simulink model "threephaseunipolar"  (Simulink 8.3)
settings: Solver=ode45  StartTime=0.0  StopTime=0.5  RelTol=1e-3
libraries: powerlib x13, simulink x3
settings Model: Creator=Singhal  LastModifiedBy=Singhal
settings OptimizationCC: ExpressionDepthLimit=2147483647
settings DebuggingCC: FcnCallInpInsideContextMsg=UseLocalSettings

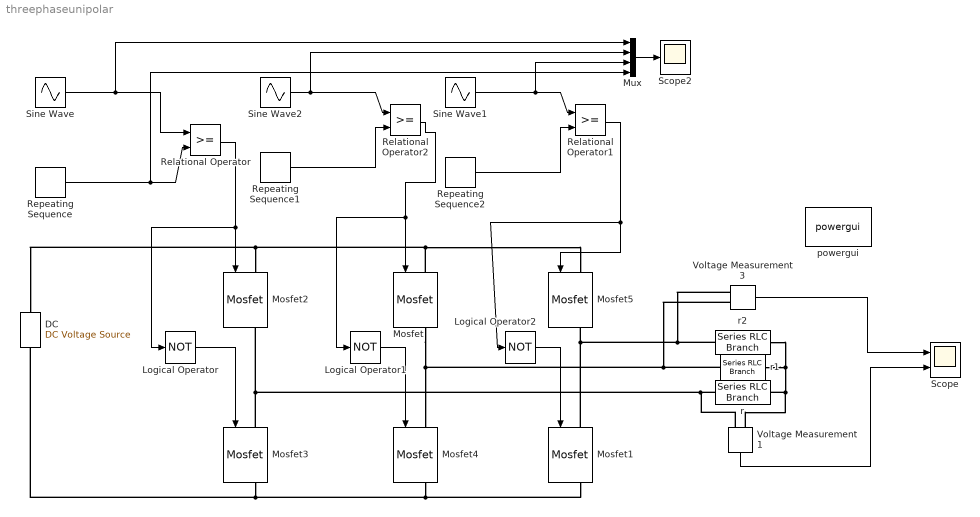
== system threephaseunipolar ==
  DC : powerlib/Electrical Sources/DC Voltage Source  Amplitude=100  Measurements=None
  Logical Operator : Logic  Operator=NOT  AllPortsSameDT=off  OutDataTypeStr=boolean
  Logical Operator1 : Logic  Operator=NOT  AllPortsSameDT=off  OutDataTypeStr=boolean
  Logical Operator2 : Logic  Operator=NOT  AllPortsSameDT=off  OutDataTypeStr=boolean
  Mosfet{,1..5} (6 alike) : powerlib/Power Electronics/Mosfet  Ron=0.1  Lon=0  Rd=0.01  Vfd=0  IC=0  Rs=1e5  Cs=inf  Measurements=on
  Mux : Mux
  Relational Operator : RelationalOperator  OutDataTypeStr=boolean
  Relational Operator1 : RelationalOperator  OutDataTypeStr=boolean
  Relational Operator2 : RelationalOperator  OutDataTypeStr=boolean
  Repeating Sequence : simulink/Sources/Repeating Sequence  rep_seq_t=[0 0.005/20 0.01/20 0.015/20 0.02/20]  rep_seq_y=[0 1 0 -1 0]
  Repeating Sequence1 : simulink/Sources/Repeating Sequence  rep_seq_t=[0 0.005/20 0.01/20 0.015/20 0.02/20]  rep_seq_y=[0 1 0 -1 0]
  Repeating Sequence2 : simulink/Sources/Repeating Sequence  rep_seq_t=[0 0.005/20 0.01/20 0.015/20 0.02/20]  rep_seq_y=[0 1 0 -1 0]
  Scope : Scope  NumInputPorts=2
      settings: YMin=-100~-5  YMax=100~5
  Scope2 : Scope
      settings: YMin=-100  YMax=100  SaveName=ScopeData2
  Sine Wave : Sin  Frequency=50*2*3.14  SampleTime=0
  Sine Wave1 : Sin  Frequency=50*2*3.14  Phase=-3.14*(4/3)  SampleTime=0
  Sine Wave2 : Sin  Frequency=50*2*3.14  Phase=-3.14*(2/3)  SampleTime=0
  Voltage Measurement1 : powerlib/Measurements/Voltage Measurement  PhasorSimulation=off  OutputType=Complex  PSBequivalent=0
  Voltage Measurement3 : powerlib/Measurements/Voltage Measurement  PhasorSimulation=off  OutputType=Complex  PSBequivalent=0
  powergui : powerlib/powergui  Priority=1  SimulationMode=Discrete  SolverType=Tustin  SampleTime=50e-6  frequency=60  SPID=off  DisableSnubberDevices=off  DisableRonSwitches=off  DisableVfSwitches=off  SwTol=0  Interpol=off  DisplayEquations=off  Ts=0  methode=off  frequencyindice=0  Pbase=100e6  ErrMax=1e-4  Iterations=50  UnitsV=kV  UnitsW=MW  FunctionMessages=off  echomessages=off  HookPort=off  EnableUseOfTLC=off  x0status=blocks  RestoreLinks=warning  ResistiveCurrentMeasurement=off  Frange=[0:2:500]  Ylog=off  Xlog=on  ShowGrid=off  save=off  variable=ZData  structure=ScopeData  ZoomFFT=on  StartTime=0.0  cycles=1  DisplayStyle=2  fundamental=50  FreqAxis=off  MaxFrequency=1000  frequencyindicesteady=1  RmsSteady=1  display=off
  r : powerlib/Elements/Series RLC Branch  LConnTagsString=__new0  RConnTagsString=__new0  BranchType=R  Resistance=1  Inductance=1e-3  SetiL0=off  InitialCurrent=0  Capacitance=1e-6  Setx0=off  InitialVoltage=0  Measurements=None
  r1 : powerlib/Elements/Series RLC Branch  LConnTagsString=__new0  RConnTagsString=__new0  BranchType=R  Resistance=1  Inductance=1e-3  SetiL0=off  InitialCurrent=0  Capacitance=1e-6  Setx0=off  InitialVoltage=0  Measurements=None
  r2 : powerlib/Elements/Series RLC Branch  LConnTagsString=__new0  RConnTagsString=__new0  BranchType=R  Resistance=1  Inductance=1e-3  SetiL0=off  InitialCurrent=0  Capacitance=1e-6  Setx0=off  InitialVoltage=0  Measurements=None
  wires:
  Sine Wave/1 -> Relational Operator/1, Mux/1
  Repeating Sequence/1 -> Relational Operator/2, Mux/4
  Logical Operator/1 -> Mosfet3/1
  Repeating Sequence2/1 -> Relational Operator1/2
  Sine Wave1/1 -> Relational Operator1/1, Mux/3
  Logical Operator1/1 -> Mosfet4/1
  Logical Operator2/1 -> Mosfet1/1
  Repeating Sequence1/1 -> Relational Operator2/2
  Sine Wave2/1 -> Relational Operator2/1, Mux/2
  Relational Operator1/1 -> Mosfet5/1, Logical Operator2/1
  Relational Operator2/1 -> Mosfet/1, Logical Operator1/1
  Relational Operator/1 -> Mosfet2/1, Logical Operator/1
  Mux/1 -> Scope2/1
  Voltage Measurement1/1 -> Scope/2
  Voltage Measurement3/1 -> Scope/1
  connections:
  Mosfet/LConn1 -- DC/RConn1 -- Mosfet2/LConn1 -- Mosfet5/LConn1
  Mosfet4/RConn1 -- DC/LConn1 -- Mosfet3/RConn1 -- Mosfet1/RConn1
  Mosfet1/LConn1 -- Voltage Measurement3/LConn1 -- r2/LConn1 -- Mosfet5/RConn1
  Mosfet/RConn1 -- r1/RConn1 -- Voltage Measurement3/LConn2 -- Mosfet4/LConn1
  Mosfet3/LConn1 -- Voltage Measurement1/LConn1 -- r/LConn1 -- Mosfet2/RConn1
  r2/RConn1 -- r1/LConn1 -- Voltage Measurement1/LConn2 -- r/RConn1
